simulink model "model_GFM_weak_18apr"  (R2024a)
settings: Solver=VariableStepAuto  StartTime=0.0  StopTime=5  RelTol=1e-3
libraries: spsThreePhaseVIMeasurementLib x4, slpidlib x4, spsThreePhaseSeriesRLCBranchLib x3, spsabctodq0Lib x3, spsThreePhaseParallelRLCLoadLib x2, eePowerMeasurement x2, spsThreePhaseBreakerLib x2, spsDCVoltageSourceLib x1, spsGroundLib x1, spsThreePhaseFaultLib x1, spsThreePhaseSourceLib x1, spsUniversalBridgeLib x1
settings Model: Creator=NAFIUNAWAR  LastModifiedBy=NAFIUNAWAR
settings DataIOCC: ReturnWorkspaceOutputs=off

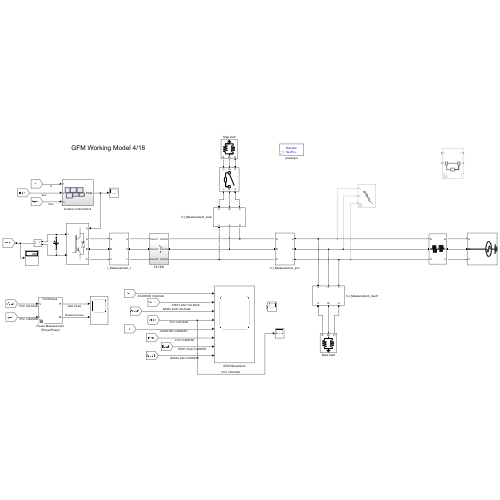
[thumbnail: Simulink's stored preview of the top-level diagram]
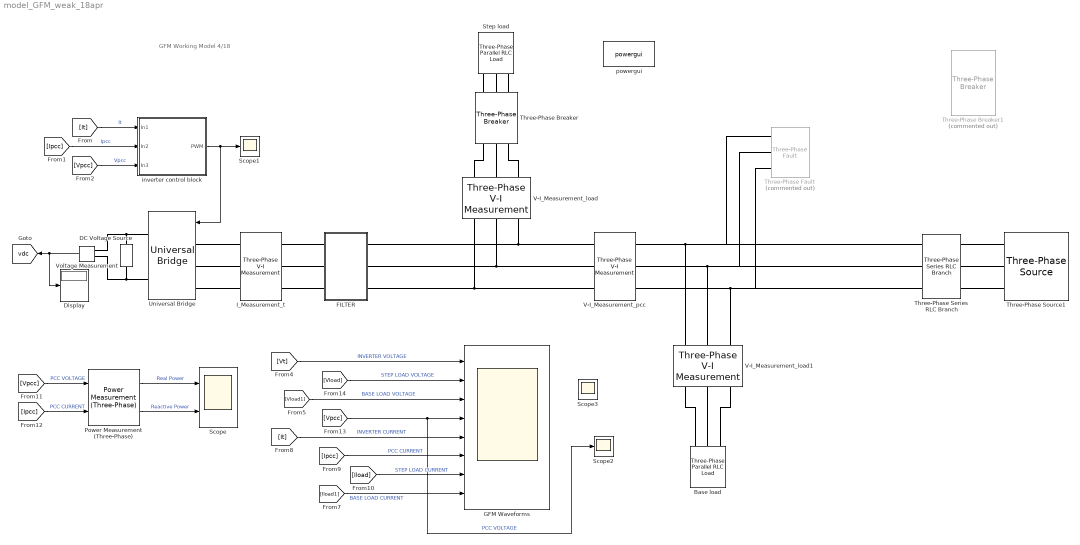
== system model_GFM_weak_18apr ==
  note: GFM Working Model 4/18
  Base load : spsThreePhaseParallelRLCLoadLib/Three-Phase Parallel RLC Load  LConnTagsString=A|B|C  Configuration=Y (grounded)  NominalVoltage=400  Vabc=[1e3 1e3 1e3]  Vabcp=[1e3 1e3 1e3]  NominalFrequency=50  UnbalancedPower=off  ActivePower=80e3  InductivePower=26.3  CapacitivePower=0  Pabc=[10e3 9e3 11e3]  QLabc=[100 90 110]  QCabc=[100 90 110]  Pabcp=[10e3 9e3 11e3]  QLabcp=[100 90 110]  QCabcp=[100 90 110]  Measurements=None  LoadType=constant Z
  DC Voltage Source : spsDCVoltageSourceLib/DC Voltage Source  Amplitude=800  Measurements=None
  Display : Display
  FILTER : Subsystem
  GFM Waveforms : Scope  NumInputPorts=8
  I_Measurement_t : spsThreePhaseVIMeasurementLib/Three-Phase V-I Measurement  VoltageMeasurement=phase-to-ground  SetLabelV=on  LabelV=Vt  Vpu=off  VpuLL=off  CurrentMeasurement=yes  SetLabelI=on  LabelI=It  Ipu=off  Pbase=100e6  Vbase=500e3  OutputType=Complex  PhasorSimulation=off  PSBequivalent=0
  Power Measurement (Three-Phase) : eePowerMeasurement/Power Measurement (Three-Phase)  LabelModeActiveChoice=Continuous  F=50  K=[0]  Seq=Positive  Ts=0
  Scope : Scope  NumInputPorts=2
  Scope1 : Scope
  Scope2 : Scope
  Scope3 : Scope
  Step load : spsThreePhaseParallelRLCLoadLib/Three-Phase Parallel RLC Load  LConnTagsString=A|B|C  Configuration=Y (grounded)  NominalVoltage=400  Vabc=[1e3 1e3 1e3]  Vabcp=[1e3 1e3 1e3]  NominalFrequency=50  UnbalancedPower=off  ActivePower=20e3  InductivePower=6.6e3  CapacitivePower=0  Pabc=[10e3 9e3 11e3]  QLabc=[100 90 110]  QCabc=[100 90 110]  Pabcp=[10e3 9e3 11e3]  QLabcp=[100 90 110]  QCabcp=[100 90 110]  Measurements=None  LoadType=constant Z
  Three-Phase Series RLC Branch : spsThreePhaseSeriesRLCBranchLib/Three-Phase Series RLC Branch  LConnTagsString=A|B|C  RConnTagsString=A|B|C  BranchType=RL  Resistance=0.05  Inductance=1.69e-3  Capacitance=1e-6  Measurements=None
  Three-Phase Breaker : spsThreePhaseBreakerLib/Three-Phase Breaker  InitialState=open  SwitchA=on  SwitchB=on  SwitchC=on  SwitchTimes=[1.5 2]  External=off  BreakerResistance=0.01  SnubberResistance=1e6  SnubberCapacitance=inf  Measurements=None
  Three-Phase Breaker1 : spsThreePhaseBreakerLib/Three-Phase Breaker  Commented=on  InitialState=closed  SwitchA=on  SwitchB=on  SwitchC=on  SwitchTimes=[3]  External=off  BreakerResistance=0.01  SnubberResistance=1e6  SnubberCapacitance=inf  Measurements=None
  Three-Phase Fault : spsThreePhaseFaultLib/Three-Phase Fault  Commented=on  InitialStates=0  FaultA=on  FaultB=on  FaultC=on  GroundFault=on  SwitchTimes=[2.1 2.3]  External=off  SwitchStatus=NaN  FaultResistance=0.001  GroundResistance=0.01  SnubberResistance=1e6  SnubberCapacitance=inf  Measurements=None
  Three-Phase Source1 : spsThreePhaseSourceLib/Three-Phase Source  InternalConnection=Yg  VoltagePhases=off  Voltage=400  PhaseAngle=0  Voltage_phases=[25e3 25e3 25e3]/sqrt(3)  PhaseAngles_phases=[0 -120 +120]  Frequency=50  NonIdealSource=off  SpecifyImpedance=off  Resistance=0.00604  Inductance=135e-6  ShortCircuitLevel=100e6  BaseVoltage=400  XRratio=7  BusType=swing  Pref=10e3  Qref=0  Prefabc=[10e3, 10e3, 10e3]  Qrefabc=[0, 0, 0]  Qmin=-inf  Qmax=inf
  Universal Bridge : spsUniversalBridgeLib/Universal Bridge  Arms=3  SnubberResistance=1e5  SnubberCapacitance=inf  Device=IGBT / Diodes  Ron=1e-3  Lon=0  ForwardVoltages="[  0  0  ]"  ForwardVoltage=0  GTOparameters=[ 10e-6 , 20e-6 ]  IGBTparameters=[ 1e-6 , 2e-6 ]  Measurements=None  Measurements_2=None  converterType=Rectifier
  V-I_Measurement_load : spsThreePhaseVIMeasurementLib/Three-Phase V-I Measurement  VoltageMeasurement=phase-to-ground  SetLabelV=on  LabelV=Vload  Vpu=on  VpuLL=off  CurrentMeasurement=yes  SetLabelI=on  LabelI=Iload  Ipu=on  Pbase=100e3  Vbase=400  OutputType=Complex  PhasorSimulation=off  PSBequivalent=0
  V-I_Measurement_load1 : spsThreePhaseVIMeasurementLib/Three-Phase V-I Measurement  VoltageMeasurement=phase-to-ground  SetLabelV=on  LabelV=Vload1  Vpu=on  VpuLL=off  CurrentMeasurement=yes  SetLabelI=on  LabelI=Iload1  Ipu=on  Pbase=100e3  Vbase=400  OutputType=Complex  PhasorSimulation=off  PSBequivalent=0
  V-I_Measurement_pcc : spsThreePhaseVIMeasurementLib/Three-Phase V-I Measurement  VoltageMeasurement=phase-to-ground  SetLabelV=on  LabelV=Vpcc  Vpu=on  VpuLL=off  CurrentMeasurement=yes  SetLabelI=on  LabelI=Ipcc  Ipu=on  Pbase=100e3  Vbase=400  OutputType=Complex  PhasorSimulation=off  PSBequivalent=0
  Voltage Measurement : spsVoltageMeasurementLib/Voltage Measurement  PhasorSimulation=off  OutputType=Complex  PSBequivalent=0
  inverter control block : Subsystem
  powergui : sps_lib/powergui  Priority=1  SimulationMode=Discrete  SampleTime=5e-5  frequency=60  Iterations=50  frequencyindice=0  Pbase=100e6  ErrMax=1e-4  UnitsV=kV  UnitsW=MW  buscounter=0  FunctionMessages=off  echomessages=off  EnableUseOfTLC=off  CurrentSourceSwitches=off  DisableSnubberDevices=off  DisableRonSwitches=off  DisableVfSwitches=off  DisplayEquations=off  AutomaticDiscreteSolvers=off  SolverType=Tustin/Backward Euler (TBE)  Interpol=off  ExternalGateDelay=off  methode=off  Ts=100  x0status=blocks  SPID=on  SwTol=0  HookPort=off  NonlinearTolerance=1e-4  nMaxIteration=100  ContinueOnMaxIteration=off  RestoreLinks=warning  ResistiveCurrentMeasurement=off  Frange=[0:2:500]  Ylog=off  Xlog=on  ShowGrid=off  save=off  variable=ZData  structure=0  ZoomFFT=off  StartTime=0.0  cycles=1  DisplayStyle=1  fundamental=60  FreqAxis=off  MaxFrequency=1000  frequencyindicesteady=1  RmsSteady=1  display=off
  tag scope: vdc=global
  wires:
  inverter control block/1(PWM) -> Universal Bridge/1, Scope1/1
  [It] -> inverter control block/1(In1)  "It"
  [Ipcc] -> inverter control block/2(In2)  "Ipcc"
  [Vpcc] -> inverter control block/3(In3)  "Vpcc"
  Voltage Measurement/1 -> Display/1, [vdc]
  [Ipcc] -> GFM Waveforms/6  "PCC CURRENT"
  [Iload] -> GFM Waveforms/7  "STEP LOAD CURRENT"
  [It] -> GFM Waveforms/5  "INVERTER CURRENT"
  [Vt] -> GFM Waveforms/1  "INVERTER VOLTAGE"
  [Iload1] -> GFM Waveforms/8  "BASE LOAD CURRENT"
  [Vpcc] -> Power Measurement (Three-Phase)/1  "PCC VOLTAGE"
  Power Measurement (Three-Phase)/1 -> Scope/1  "Real Power"
  Power Measurement (Three-Phase)/2 -> Scope/2  "Reactive Power"
  [Ipcc] -> Power Measurement (Three-Phase)/2  "PCC CURRENT"
  [Vload] -> GFM Waveforms/2  "STEP LOAD VOLTAGE"
  [Vload1] -> GFM Waveforms/3  "BASE LOAD VOLTAGE"
  [Vpcc] -> Scope2/1, GFM Waveforms/4  "PCC VOLTAGE"
  connections:
  Universal Bridge/RConn1 -- Voltage Measurement/LConn1 -- DC Voltage Source/RConn1
  DC Voltage Source/LConn1 -- Voltage Measurement/LConn2 -- Universal Bridge/RConn2
  I_Measurement_t/LConn1 -- Universal Bridge/LConn1
  Universal Bridge/LConn2 -- I_Measurement_t/LConn2
  Universal Bridge/LConn3 -- I_Measurement_t/LConn3
  V-I_Measurement_load/RConn2 -- V-I_Measurement_pcc/LConn2 -- FILTER/RConn2
  V-I_Measurement_pcc/RConn1 -- Three-Phase Series RLC Branch/LConn1 -- Three-Phase Fault/LConn1 -- V-I_Measurement_load1/RConn1
  V-I_Measurement_pcc/RConn2 -- Three-Phase Fault/LConn2 -- Three-Phase Series RLC Branch/LConn2 -- V-I_Measurement_load1/RConn2
  V-I_Measurement_pcc/RConn3 -- Three-Phase Series RLC Branch/LConn3 -- Three-Phase Fault/LConn3 -- V-I_Measurement_load1/RConn3
  Step load/LConn1 -- Three-Phase Breaker/LConn3
  Three-Phase Breaker/LConn2 -- Step load/LConn2
  Step load/LConn3 -- Three-Phase Breaker/LConn1
  V-I_Measurement_load/LConn2 -- Three-Phase Breaker/RConn2
  V-I_Measurement_load/LConn1 -- Three-Phase Breaker/RConn1
  Three-Phase Breaker/RConn3 -- V-I_Measurement_load/LConn3
  Base load/LConn3 -- V-I_Measurement_load1/LConn3
  Base load/LConn1 -- V-I_Measurement_load1/LConn1
  Base load/LConn2 -- V-I_Measurement_load1/LConn2
  V-I_Measurement_load/RConn3 -- V-I_Measurement_pcc/LConn3 -- FILTER/RConn3
  V-I_Measurement_load/RConn1 -- V-I_Measurement_pcc/LConn1 -- FILTER/RConn1
  FILTER/LConn1 -- I_Measurement_t/RConn1
  FILTER/LConn2 -- I_Measurement_t/RConn2
  FILTER/LConn3 -- I_Measurement_t/RConn3
  Three-Phase Series RLC Branch/RConn3 -- Three-Phase Source1/RConn3
  Three-Phase Series RLC Branch/RConn1 -- Three-Phase Source1/RConn1
  Three-Phase Series RLC Branch/RConn2 -- Three-Phase Source1/RConn2

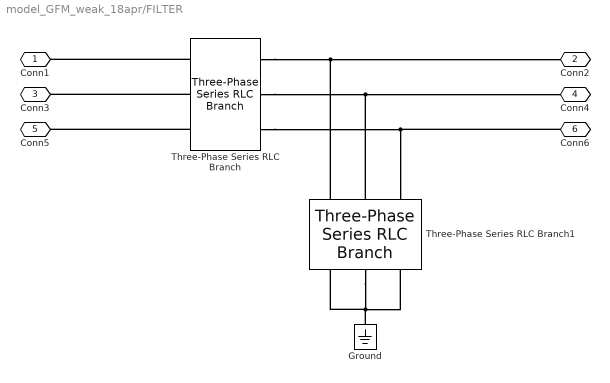
== system model_GFM_weak_18apr/FILTER ==
  Ground : spsGroundLib/Ground  LConnTagsString=a
  Three-Phase Series RLC Branch : spsThreePhaseSeriesRLCBranchLib/Three-Phase Series RLC Branch  LConnTagsString=A|B|C  RConnTagsString=A|B|C  BranchType=RL  Resistance=10e-3  Inductance=95e-6  Capacitance=1e-6  Measurements=None
  Three-Phase Series RLC Branch1 : spsThreePhaseSeriesRLCBranchLib/Three-Phase Series RLC Branch  LConnTagsString=A|B|C  RConnTagsString=A|B|C  BranchType=C  Resistance=10e-3  Inductance=95e-6  Capacitance=1e-03  Measurements=None
  Conn1 : PMIOPort  Side=Left
  Conn2 : PMIOPort  Port=2  Side=Right
  Conn3 : PMIOPort  Port=3  Side=Left
  Conn4 : PMIOPort  Port=4  Side=Right
  Conn5 : PMIOPort  Port=5  Side=Left
  Conn6 : PMIOPort  Port=6  Side=Right
  connections:
  Three-Phase Series RLC Branch/LConn3 -- Conn5/RConn1
  Three-Phase Series RLC Branch/RConn1 -- Conn2/RConn1 -- Three-Phase Series RLC Branch1/LConn1
  Ground/LConn1 -- Three-Phase Series RLC Branch1/RConn3 -- Three-Phase Series RLC Branch1/RConn1 -- Three-Phase Series RLC Branch1/RConn2
  Three-Phase Series RLC Branch1/LConn2 -- Conn4/RConn1 -- Three-Phase Series RLC Branch/RConn2
  Three-Phase Series RLC Branch/RConn3 -- Conn6/RConn1 -- Three-Phase Series RLC Branch1/LConn3
  Three-Phase Series RLC Branch/LConn1 -- Conn1/RConn1
  Three-Phase Series RLC Branch/LConn2 -- Conn3/RConn1

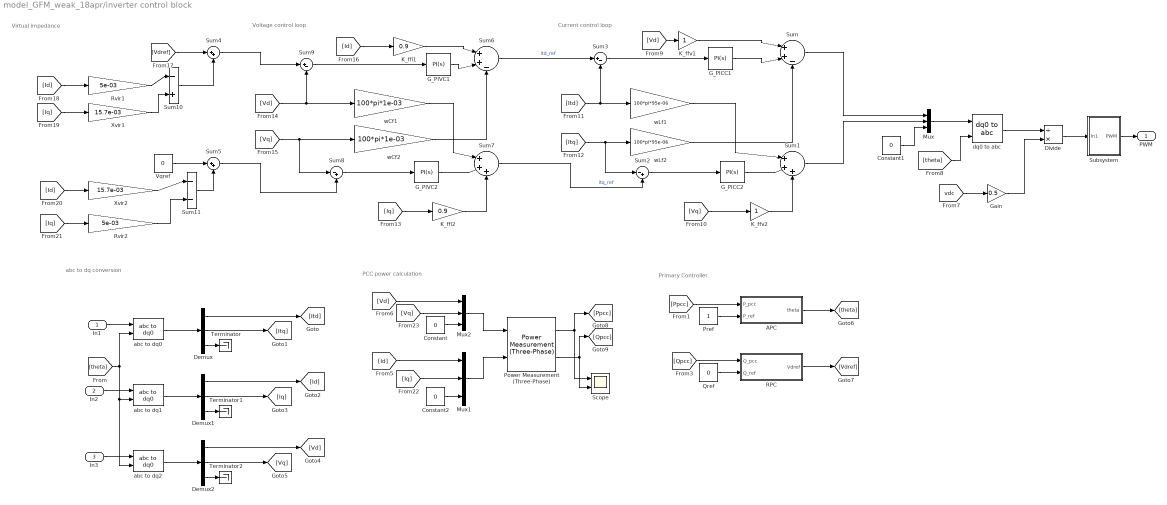
== system model_GFM_weak_18apr/inverter control block ==
  note: abc to dq conversion
  note: PCC power calculation
  note: Primary Controller
  note: Virtual impedance
  note: Current control loop
  note: Voltage control loop
  In1 : Inport
  In2 : Inport  Port=2
  In3 : Inport  Port=3
  APC : Subsystem
  Constant : Constant  Value=0
  Constant1 : Constant  Value=0
  Constant2 : Constant  Value=0
  Demux : Demux  Outputs=3
  Demux1 : Demux  Outputs=3
  Demux2 : Demux  Outputs=3
  Divide : Product  Inputs=/*
  G_PICC1 : slpidlib/PID Controller  Controller=PI  Form=Parallel  TimeDomain=Continuous-time  UseExternalTs=off  SampleTime=-1  IntegratorMethod=Forward Euler  FilterMethod=Forward Euler  ControllerParametersSource=internal  P=0.1425  I=15  UseKiTs=off  D=0  UseExternalDerivativeSource=off  N=100  UseFilter=on  TunerSelectOption=Transfer Function Based (PID Tuner App)  InitialConditionSource=internal  InitialConditionForIntegrator=0  InitialConditionForFilter=0  DifferentiatorICPrevScaledInput=0  ExternalReset=none  TrackingMode=off  Kt=1  LimitOutput=off  SatLimitsSource=internal  UpperSaturationLimit=inf  LowerSaturationLimit=-inf  LinearizeAsGain=on  AntiWindupMode=none  Kb=1  LimitIntegrator=off  UpperIntegratorSaturationLimit=inf  LowerIntegratorSaturationLimit=-inf  POutMin=[]  POutMax=[]  IOutMin=[]  IOutMax=[]  DOutMin=[]  DOutMax=[]  NOutMin=[]  NOutMax=[]  SumOutMin=[]  SumOutMax=[]  SaturationOutMin=[]  SaturationOutMax=[]  PParamMin=[]  PParamMax=[]  IParamMin=[]  IParamMax=[]  DParamMin=[]  DParamMax=[]  NParamMin=[]  NParamMax=[]  KbParamMin=[]  KbParamMax=[]  KtParamMin=[]  KtParamMax=[]  KbOutMin=[]  KbOutMax=[]  KtOutMin=[]  KtOutMax=[]  IntegratorOutMin=[]  IntegratorOutMax=[]  FilterOutMin=[]  FilterOutMax=[]  SumI1OutMin=[]  SumI1OutMax=[]  SumI2OutMin=[]  SumI2OutMax=[]  SumI3OutMin=[]  SumI3OutMax=[]  SumI4OutMin=[]  SumI4OutMax=[]  SumDOutMin=[]  SumDOutMax=[]  DifferentiatorOutMin=[]  DifferentiatorOutMax=[]  FilterDiffOutCoefMin=[]  FilterDiffOutCoefMax=[]  ReciprocalOutMin=[]  ReciprocalOutMax=[]  SumDenOutMin=[]  SumDenOutMax=[]  SumNumOutMin=[]  SumNumOutMax=[]  DivideOutMin=[]  DivideOutMax=[]  UdiffTsProdOutMin=[]  UdiffTsProdOutMax=[]  NTsProdOutMin=[]  NTsProdOutMax=[]  UintegralTsProdOutMin=[]  UintegralTsProdOutMax=[]  UngainTsProdOutMin=[]  UngainTsProdOutMax=[]  ClampingZeroOutDataTypeStr=Inherit: Inherit via back propagation  ClampingZeroOutMin=[]  ClampingZeroOutMax=[]  FilterDenConstantOutDataTypeStr=Inherit: Inherit via back propagation  FilterDenConstantOutMin=[]  FilterDenConstantOutMax=[]  PCopyOutDataTypeStr=Inherit: Inherit via back propagation  PCopyOutMin=[]  PCopyOutMax=[]  NCopyOutDataTypeStr=Inherit: Inherit via back propagation  NCopyOutMin=[]  NCopyOutMax=[]  IntegratorContinuousStateAttributes=''  IntegratorStateMustResolveToSignalObject=off  IntegratorRTWStateStorageClass=Auto  FilterContinuousStateAttributes=''  FilterStateMustResolveToSignalObject=off  FilterRTWStateStorageClass=Auto  ParallelPVariant=InternalParameters  IdealPVariant=Disabled  IVariant=InternalParameters  DVariant=Disabled  IntegratorVariant=Continuous  SatVariant=Disabled  AWVariant=Passthrough  PCopyVariant=Disabled  TRVariant=Disabled  FdbkBlocksVariant=Forward  IdealPFdbkVariant=Disabled  SatFdbkVariant=Disabled  DerivativeFilterVariant=Disabled  NVariant=Disabled  NCopyVariant=Disabled_SignalSpec  FilterICVariant=Disabled  IntegratorICVariant=InternalICs  ExternalResetVariant=Disabled  TRSumVariant=Passthrough  SumFdbkVariant=Disabled  SumVariant=Sum_PI  TsampFilterVariant=InternalTs  TsampNgainVariant=Passthrough  TsampIntegralVariant=Disabled_SignalSpec  ExternalSaturationOutDataTypeStr=Inherit: Same as second input  DerivativeSourceVariant=Disabled
  G_PICC2 : slpidlib/PID Controller  Controller=PI  Form=Parallel  TimeDomain=Continuous-time  UseExternalTs=off  SampleTime=-1  IntegratorMethod=Forward Euler  FilterMethod=Forward Euler  ControllerParametersSource=internal  P=0.1425  I=15  UseKiTs=off  D=0  UseExternalDerivativeSource=off  N=100  UseFilter=on  TunerSelectOption=Transfer Function Based (PID Tuner App)  InitialConditionSource=internal  InitialConditionForIntegrator=0  InitialConditionForFilter=0  DifferentiatorICPrevScaledInput=0  ExternalReset=none  TrackingMode=off  Kt=1  LimitOutput=off  SatLimitsSource=internal  UpperSaturationLimit=inf  LowerSaturationLimit=-inf  LinearizeAsGain=on  AntiWindupMode=none  Kb=1  LimitIntegrator=off  UpperIntegratorSaturationLimit=inf  LowerIntegratorSaturationLimit=-inf  POutMin=[]  POutMax=[]  IOutMin=[]  IOutMax=[]  DOutMin=[]  DOutMax=[]  NOutMin=[]  NOutMax=[]  SumOutMin=[]  SumOutMax=[]  SaturationOutMin=[]  SaturationOutMax=[]  PParamMin=[]  PParamMax=[]  IParamMin=[]  IParamMax=[]  DParamMin=[]  DParamMax=[]  NParamMin=[]  NParamMax=[]  KbParamMin=[]  KbParamMax=[]  KtParamMin=[]  KtParamMax=[]  KbOutMin=[]  KbOutMax=[]  KtOutMin=[]  KtOutMax=[]  IntegratorOutMin=[]  IntegratorOutMax=[]  FilterOutMin=[]  FilterOutMax=[]  SumI1OutMin=[]  SumI1OutMax=[]  SumI2OutMin=[]  SumI2OutMax=[]  SumI3OutMin=[]  SumI3OutMax=[]  SumI4OutMin=[]  SumI4OutMax=[]  SumDOutMin=[]  SumDOutMax=[]  DifferentiatorOutMin=[]  DifferentiatorOutMax=[]  FilterDiffOutCoefMin=[]  FilterDiffOutCoefMax=[]  ReciprocalOutMin=[]  ReciprocalOutMax=[]  SumDenOutMin=[]  SumDenOutMax=[]  SumNumOutMin=[]  SumNumOutMax=[]  DivideOutMin=[]  DivideOutMax=[]  UdiffTsProdOutMin=[]  UdiffTsProdOutMax=[]  NTsProdOutMin=[]  NTsProdOutMax=[]  UintegralTsProdOutMin=[]  UintegralTsProdOutMax=[]  UngainTsProdOutMin=[]  UngainTsProdOutMax=[]  ClampingZeroOutDataTypeStr=Inherit: Inherit via back propagation  ClampingZeroOutMin=[]  ClampingZeroOutMax=[]  FilterDenConstantOutDataTypeStr=Inherit: Inherit via back propagation  FilterDenConstantOutMin=[]  FilterDenConstantOutMax=[]  PCopyOutDataTypeStr=Inherit: Inherit via back propagation  PCopyOutMin=[]  PCopyOutMax=[]  NCopyOutDataTypeStr=Inherit: Inherit via back propagation  NCopyOutMin=[]  NCopyOutMax=[]  IntegratorContinuousStateAttributes=''  IntegratorStateMustResolveToSignalObject=off  IntegratorRTWStateStorageClass=Auto  FilterContinuousStateAttributes=''  FilterStateMustResolveToSignalObject=off  FilterRTWStateStorageClass=Auto  ParallelPVariant=InternalParameters  IdealPVariant=Disabled  IVariant=InternalParameters  DVariant=Disabled  IntegratorVariant=Continuous  SatVariant=Disabled  AWVariant=Passthrough  PCopyVariant=Disabled  TRVariant=Disabled  FdbkBlocksVariant=Forward  IdealPFdbkVariant=Disabled  SatFdbkVariant=Disabled  DerivativeFilterVariant=Disabled  NVariant=Disabled  NCopyVariant=Disabled_SignalSpec  FilterICVariant=Disabled  IntegratorICVariant=InternalICs  ExternalResetVariant=Disabled  TRSumVariant=Passthrough  SumFdbkVariant=Disabled  SumVariant=Sum_PI  TsampFilterVariant=InternalTs  TsampNgainVariant=Passthrough  TsampIntegralVariant=Disabled_SignalSpec  ExternalSaturationOutDataTypeStr=Inherit: Same as second input  DerivativeSourceVariant=Disabled
  G_PIVC1 : slpidlib/PID Controller  Controller=PI  Form=Parallel  TimeDomain=Continuous-time  UseExternalTs=off  SampleTime=-1  IntegratorMethod=Forward Euler  FilterMethod=Forward Euler  ControllerParametersSource=internal  P=14.25  I=1500  UseKiTs=off  D=0  UseExternalDerivativeSource=off  N=100  UseFilter=on  TunerSelectOption=Transfer Function Based (PID Tuner App)  InitialConditionSource=internal  InitialConditionForIntegrator=0  InitialConditionForFilter=0  DifferentiatorICPrevScaledInput=0  ExternalReset=none  TrackingMode=off  Kt=1  LimitOutput=off  SatLimitsSource=internal  UpperSaturationLimit=inf  LowerSaturationLimit=-inf  LinearizeAsGain=on  AntiWindupMode=none  Kb=1  LimitIntegrator=off  UpperIntegratorSaturationLimit=inf  LowerIntegratorSaturationLimit=-inf  POutMin=[]  POutMax=[]  IOutMin=[]  IOutMax=[]  DOutMin=[]  DOutMax=[]  NOutMin=[]  NOutMax=[]  SumOutMin=[]  SumOutMax=[]  SaturationOutMin=[]  SaturationOutMax=[]  PParamMin=[]  PParamMax=[]  IParamMin=[]  IParamMax=[]  DParamMin=[]  DParamMax=[]  NParamMin=[]  NParamMax=[]  KbParamMin=[]  KbParamMax=[]  KtParamMin=[]  KtParamMax=[]  KbOutMin=[]  KbOutMax=[]  KtOutMin=[]  KtOutMax=[]  IntegratorOutMin=[]  IntegratorOutMax=[]  FilterOutMin=[]  FilterOutMax=[]  SumI1OutMin=[]  SumI1OutMax=[]  SumI2OutMin=[]  SumI2OutMax=[]  SumI3OutMin=[]  SumI3OutMax=[]  SumI4OutMin=[]  SumI4OutMax=[]  SumDOutMin=[]  SumDOutMax=[]  DifferentiatorOutMin=[]  DifferentiatorOutMax=[]  FilterDiffOutCoefMin=[]  FilterDiffOutCoefMax=[]  ReciprocalOutMin=[]  ReciprocalOutMax=[]  SumDenOutMin=[]  SumDenOutMax=[]  SumNumOutMin=[]  SumNumOutMax=[]  DivideOutMin=[]  DivideOutMax=[]  UdiffTsProdOutMin=[]  UdiffTsProdOutMax=[]  NTsProdOutMin=[]  NTsProdOutMax=[]  UintegralTsProdOutMin=[]  UintegralTsProdOutMax=[]  UngainTsProdOutMin=[]  UngainTsProdOutMax=[]  ClampingZeroOutDataTypeStr=Inherit: Inherit via back propagation  ClampingZeroOutMin=[]  ClampingZeroOutMax=[]  FilterDenConstantOutDataTypeStr=Inherit: Inherit via back propagation  FilterDenConstantOutMin=[]  FilterDenConstantOutMax=[]  PCopyOutDataTypeStr=Inherit: Inherit via back propagation  PCopyOutMin=[]  PCopyOutMax=[]  NCopyOutDataTypeStr=Inherit: Inherit via back propagation  NCopyOutMin=[]  NCopyOutMax=[]  IntegratorContinuousStateAttributes=''  IntegratorStateMustResolveToSignalObject=off  IntegratorRTWStateStorageClass=Auto  FilterContinuousStateAttributes=''  FilterStateMustResolveToSignalObject=off  FilterRTWStateStorageClass=Auto  ParallelPVariant=InternalParameters  IdealPVariant=Disabled  IVariant=InternalParameters  DVariant=Disabled  IntegratorVariant=Continuous  SatVariant=Disabled  AWVariant=Passthrough  PCopyVariant=Disabled  TRVariant=Disabled  FdbkBlocksVariant=Forward  IdealPFdbkVariant=Disabled  SatFdbkVariant=Disabled  DerivativeFilterVariant=Disabled  NVariant=Disabled  NCopyVariant=Disabled_SignalSpec  FilterICVariant=Disabled  IntegratorICVariant=InternalICs  ExternalResetVariant=Disabled  TRSumVariant=Passthrough  SumFdbkVariant=Disabled  SumVariant=Sum_PI  TsampFilterVariant=InternalTs  TsampNgainVariant=Passthrough  TsampIntegralVariant=Disabled_SignalSpec  ExternalSaturationOutDataTypeStr=Inherit: Same as second input  DerivativeSourceVariant=Disabled
  G_PIVC2 : slpidlib/PID Controller  Controller=PI  Form=Parallel  TimeDomain=Continuous-time  UseExternalTs=off  SampleTime=-1  IntegratorMethod=Forward Euler  FilterMethod=Forward Euler  ControllerParametersSource=internal  P=14.25  I=1500  UseKiTs=off  D=0  UseExternalDerivativeSource=off  N=100  UseFilter=on  TunerSelectOption=Transfer Function Based (PID Tuner App)  InitialConditionSource=internal  InitialConditionForIntegrator=0  InitialConditionForFilter=0  DifferentiatorICPrevScaledInput=0  ExternalReset=none  TrackingMode=off  Kt=1  LimitOutput=off  SatLimitsSource=internal  UpperSaturationLimit=inf  LowerSaturationLimit=-inf  LinearizeAsGain=on  AntiWindupMode=none  Kb=1  LimitIntegrator=off  UpperIntegratorSaturationLimit=inf  LowerIntegratorSaturationLimit=-inf  POutMin=[]  POutMax=[]  IOutMin=[]  IOutMax=[]  DOutMin=[]  DOutMax=[]  NOutMin=[]  NOutMax=[]  SumOutMin=[]  SumOutMax=[]  SaturationOutMin=[]  SaturationOutMax=[]  PParamMin=[]  PParamMax=[]  IParamMin=[]  IParamMax=[]  DParamMin=[]  DParamMax=[]  NParamMin=[]  NParamMax=[]  KbParamMin=[]  KbParamMax=[]  KtParamMin=[]  KtParamMax=[]  KbOutMin=[]  KbOutMax=[]  KtOutMin=[]  KtOutMax=[]  IntegratorOutMin=[]  IntegratorOutMax=[]  FilterOutMin=[]  FilterOutMax=[]  SumI1OutMin=[]  SumI1OutMax=[]  SumI2OutMin=[]  SumI2OutMax=[]  SumI3OutMin=[]  SumI3OutMax=[]  SumI4OutMin=[]  SumI4OutMax=[]  SumDOutMin=[]  SumDOutMax=[]  DifferentiatorOutMin=[]  DifferentiatorOutMax=[]  FilterDiffOutCoefMin=[]  FilterDiffOutCoefMax=[]  ReciprocalOutMin=[]  ReciprocalOutMax=[]  SumDenOutMin=[]  SumDenOutMax=[]  SumNumOutMin=[]  SumNumOutMax=[]  DivideOutMin=[]  DivideOutMax=[]  UdiffTsProdOutMin=[]  UdiffTsProdOutMax=[]  NTsProdOutMin=[]  NTsProdOutMax=[]  UintegralTsProdOutMin=[]  UintegralTsProdOutMax=[]  UngainTsProdOutMin=[]  UngainTsProdOutMax=[]  ClampingZeroOutDataTypeStr=Inherit: Inherit via back propagation  ClampingZeroOutMin=[]  ClampingZeroOutMax=[]  FilterDenConstantOutDataTypeStr=Inherit: Inherit via back propagation  FilterDenConstantOutMin=[]  FilterDenConstantOutMax=[]  PCopyOutDataTypeStr=Inherit: Inherit via back propagation  PCopyOutMin=[]  PCopyOutMax=[]  NCopyOutDataTypeStr=Inherit: Inherit via back propagation  NCopyOutMin=[]  NCopyOutMax=[]  IntegratorContinuousStateAttributes=''  IntegratorStateMustResolveToSignalObject=off  IntegratorRTWStateStorageClass=Auto  FilterContinuousStateAttributes=''  FilterStateMustResolveToSignalObject=off  FilterRTWStateStorageClass=Auto  ParallelPVariant=InternalParameters  IdealPVariant=Disabled  IVariant=InternalParameters  DVariant=Disabled  IntegratorVariant=Continuous  SatVariant=Disabled  AWVariant=Passthrough  PCopyVariant=Disabled  TRVariant=Disabled  FdbkBlocksVariant=Forward  IdealPFdbkVariant=Disabled  SatFdbkVariant=Disabled  DerivativeFilterVariant=Disabled  NVariant=Disabled  NCopyVariant=Disabled_SignalSpec  FilterICVariant=Disabled  IntegratorICVariant=InternalICs  ExternalResetVariant=Disabled  TRSumVariant=Passthrough  SumFdbkVariant=Disabled  SumVariant=Sum_PI  TsampFilterVariant=InternalTs  TsampNgainVariant=Passthrough  TsampIntegralVariant=Disabled_SignalSpec  ExternalSaturationOutDataTypeStr=Inherit: Same as second input  DerivativeSourceVariant=Disabled
  Gain : Gain  Gain=0.5
  K_ffi1 : Gain  Gain=0.9
  K_ffi2 : Gain  Gain=0.9
  K_ffv1 : Gain
  K_ffv2 : Gain
  Mux : Mux  Inputs=3
  Mux1 : Mux  Inputs=3
  Mux2 : Mux  Inputs=3
  Power Measurement (Three-Phase) : eePowerMeasurement/Power Measurement (Three-Phase)  LabelModeActiveChoice=Continuous  F=50  K=[1]  Seq=Positive  Ts=0
  Pref : Constant
  Qref : Constant  Value=0
  RPC : Subsystem
  Rvir1 : Gain  Gain=5e-03
  Rvir2 : Gain  Gain=5e-03
  Scope : Scope  NumInputPorts=2
  Subsystem : Subsystem
  Sum : Sum  Inputs=|++-
  Sum1 : Sum  Inputs=|+++
  Sum10 : Sum  Inputs=|-+
  Sum11 : Sum  Inputs=|--
  Sum2 : Sum  Inputs=|-+
  Sum3 : Sum  Inputs=|+-
  Sum4 : Sum  Inputs=|++
  Sum5 : Sum  Inputs=|++
  Sum6 : Sum  Inputs=|++-
  Sum7 : Sum  Inputs=|+++
  Sum8 : Sum  Inputs=|-+
  Sum9 : Sum  Inputs=|+-
  Terminator : Terminator
  Terminator1 : Terminator
  Terminator2 : Terminator
  Vqref : Constant  Value=0
  Xvir1 : Gain  Gain=15.7e-03
  Xvir2 : Gain  Gain=15.7e-03
  abc to dq0 : spsabctodq0Lib/abc to dq0  Alignment=90 degrees behind phase A axis
  abc to dq1 : spsabctodq0Lib/abc to dq0  Alignment=90 degrees behind phase A axis
  abc to dq2 : spsabctodq0Lib/abc to dq0  Alignment=90 degrees behind phase A axis
  dq0 to abc : spsdq0toabcLib/dq0 to abc  Alignment=90 degrees behind phase A axis
  wCf1 : Gain  Gain=100*pi*1e-03
  wCf2 : Gain  Gain=100*pi*1e-03
  wLf1 : Gain  Gain=100*pi*95e-06
  wLf2 : Gain  Gain=100*pi*95e-06
  PWM : Outport
  wires:
  In1/1 -> abc to dq0/1
  In2/1 -> abc to dq1/1
  In3/1 -> abc to dq2/1
  abc to dq0/1 -> Demux/1
  Demux/3 -> Terminator/1
  Demux1/3 -> Terminator1/1
  abc to dq1/1 -> Demux1/1
  Demux2/3 -> Terminator2/1
  abc to dq2/1 -> Demux2/1
  Demux/1 -> [Itd]
  Demux/2 -> [Itq]
  Demux1/2 -> [Iq]
  Demux1/1 -> [Id]
  Demux2/2 -> [Vq]
  Demux2/1 -> [Vd]
  [theta] -> abc to dq2/2, abc to dq1/2, abc to dq0/2
  APC/1(theta) -> [theta]
  RPC/1(Vdref) -> [Vdref]
  [Ppcc] -> APC/1(P_pcc)
  Pref/1 -> APC/2(P_ref)
  [Qpcc] -> RPC/1(Q_pcc)
  Qref/1 -> RPC/2(Q_ref)
  Power Measurement (Three-Phase)/1 -> [Ppcc], Scope/1
  Power Measurement (Three-Phase)/2 -> [Qpcc], Scope/2
  [theta] -> dq0 to abc/2
  Mux/1 -> dq0 to abc/1
  Sum/1 -> Mux/1
  Sum1/1 -> Mux/2
  G_PICC1/1 -> Sum/2
  G_PICC2/1 -> Sum1/2
  K_ffv2/1 -> Sum1/3
  K_ffv1/1 -> Sum/1
  [Vd] -> K_ffv1/1
  [Vq] -> K_ffv2/1
  Sum3/1 -> G_PICC1/1
  Sum2/1 -> G_PICC2/1
  [Itd] -> Sum3/2, wLf1/1
  [Itq] -> Sum2/1, wLf2/1
  wLf1/1 -> Sum1/1
  wLf2/1 -> Sum/3
  wCf2/1 -> Sum6/3
  wCf1/1 -> Sum7/1
  [Vq] -> Sum8/1, wCf2/1
  [Vd] -> Sum9/2, wCf1/1
  Sum8/1 -> G_PIVC2/1
  Sum9/1 -> G_PIVC1/1
  [Iq] -> K_ffi2/1
  [Id] -> K_ffi1/1
  K_ffi1/1 -> Sum6/1
  K_ffi2/1 -> Sum7/3
  G_PIVC2/1 -> Sum7/2
  G_PIVC1/1 -> Sum6/2
  Sum6/1 -> Sum3/1  "itd_ref"
  Sum7/1 -> Sum2/2  "itq_ref"
  Sum4/1 -> Sum9/1
  Sum5/1 -> Sum8/2
  [Vdref] -> Sum4/1
  Vqref/1 -> Sum5/1
  Sum10/1 -> Sum4/2
  Sum11/1 -> Sum5/2
  Xvir2/1 -> Sum11/1
  Rvir2/1 -> Sum11/2
  Rvir1/1 -> Sum10/1
  Xvir1/1 -> Sum10/2
  [Id] -> Rvir1/1
  [Iq] -> Xvir1/1
  [Id] -> Xvir2/1
  [Iq] -> Rvir2/1
  [Id] -> Mux1/1
  [Iq] -> Mux1/2
  Mux1/1 -> Power Measurement (Three-Phase)/2
  Mux2/1 -> Power Measurement (Three-Phase)/1
  [Vd] -> Mux2/1
  [Vq] -> Mux2/2
  Constant1/1 -> Mux/3
  Divide/1 -> Subsystem/1(In1)
  Subsystem/1(PWM) -> PWM/1
  Constant2/1 -> Mux1/3
  Constant/1 -> Mux2/3
  [vdc] -> Gain/1
  Gain/1 -> Divide/2
  dq0 to abc/1 -> Divide/1

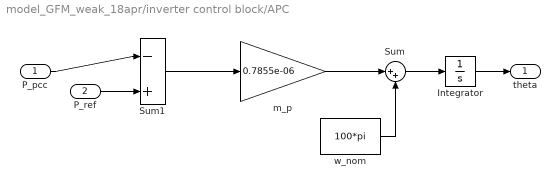
== system model_GFM_weak_18apr/inverter control block/APC ==
  P_pcc : Inport
  P_ref : Inport  Port=2
  Integrator : Integrator
  Sum : Sum  Inputs=|++
  Sum1 : Sum  Inputs=|-+
  m_p : Gain  Gain=0.7855e-06
  w_nom : Constant  Value=100*pi
  theta : Outport
  wires:
  P_ref/1 -> Sum1/2
  P_pcc/1 -> Sum1/1
  Sum1/1 -> m_p/1
  m_p/1 -> Sum/1
  w_nom/1 -> Sum/2
  Integrator/1 -> theta/1
  Sum/1 -> Integrator/1

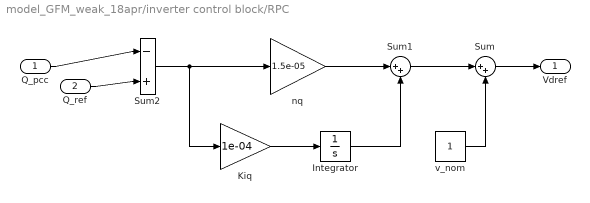
== system model_GFM_weak_18apr/inverter control block/RPC ==
  Q_pcc : Inport
  Q_ref : Inport  Port=2
  Integrator : Integrator
  Kiq : Gain  Gain=1e-04
  Sum : Sum  Inputs=|++
  Sum1 : Sum  Inputs=|++
  Sum2 : Sum  Inputs=|-+
  nq : Gain  Gain=1.5e-05
  v_nom : Constant
  Vdref : Outport
  wires:
  Sum/1 -> Vdref/1
  Sum1/1 -> Sum/1
  Q_pcc/1 -> Sum2/1
  Q_ref/1 -> Sum2/2
  nq/1 -> Sum1/1
  Sum2/1 -> Kiq/1, nq/1
  v_nom/1 -> Sum/2
  Kiq/1 -> Integrator/1
  Integrator/1 -> Sum1/2

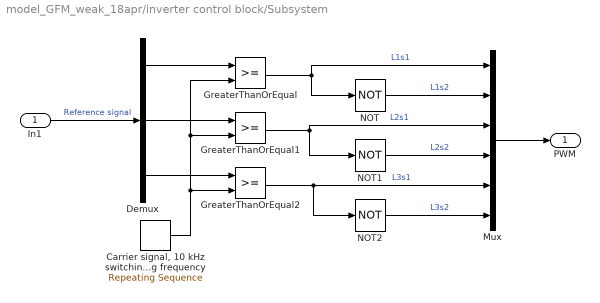
== system model_GFM_weak_18apr/inverter control block/Subsystem ==
  In1 : Inport
  "Carrier signal, 10 kHz switching frequency" : simulink/Sources/Repeating Sequence  rep_seq_t=[0 0.00005 0.001]  rep_seq_y=[-1 1 -1]
  Demux : Demux  Outputs=3
  GreaterThanOrEqual : RelationalOperator  OutDataTypeStr=boolean  RndMeth=Simplest  InputSameDT=off
  GreaterThanOrEqual1 : RelationalOperator  OutDataTypeStr=boolean  RndMeth=Simplest  InputSameDT=off
  GreaterThanOrEqual2 : RelationalOperator  OutDataTypeStr=boolean  RndMeth=Simplest  InputSameDT=off
  Mux : Mux  Inputs=6
  NOT : Logic  Operator=NOT  IconShape=distinctive  AllPortsSameDT=off  OutDataTypeStr=boolean
  NOT1 : Logic  Operator=NOT  IconShape=distinctive  AllPortsSameDT=off  OutDataTypeStr=boolean
  NOT2 : Logic  Operator=NOT  IconShape=distinctive  AllPortsSameDT=off  OutDataTypeStr=boolean
  PWM : Outport
  wires:
  GreaterThanOrEqual2/1 -> NOT2/1, Mux/5  "L3s1"
  Mux/1 -> PWM/1
  NOT2/1 -> Mux/6  "L3s2"
  GreaterThanOrEqual/1 -> Mux/1, NOT/1  "L1s1"
  In1/1 -> Demux/1  "Reference signal"
  GreaterThanOrEqual1/1 -> NOT1/1, Mux/3  "L2s1"
  "Carrier signal, 10 kHz switching frequency"/1 -> GreaterThanOrEqual/2, GreaterThanOrEqual1/2, GreaterThanOrEqual2/2
  Demux/2 -> GreaterThanOrEqual1/1
  NOT1/1 -> Mux/4  "L2s2"
  NOT/1 -> Mux/2  "L1s2"
  Demux/3 -> GreaterThanOrEqual2/1
  Demux/1 -> GreaterThanOrEqual/1
